simulink library "inverter_loop_pump_and_fan_PWM_LVLibrary"  (R2020a)
settings: Solver=ode45  StartTime=0.0  StopTime=10.0  RelTol=1e-3  EnableMultiTasking=on
undefined symbols (not defined in the file): CR
libraries: simulink x6
settings Model: Creator=aldernl  LastModifiedBy=Harjot
settings DataIOCC: LimitDataPoints=on
settings OptimizationCC: LifeSpan=inf
settings DebuggingCC: AllowSymbolicDim=off  SFUnexpectedBacktrackingDiag=warning  SFNoUnconditionalDefaultTransitionDiag=warning  ArithmeticOperatorsInVariantConditions=warning
settings SFSimCC: SimUseLocalCustomCode=off  CustomCodeUndefinedFunction=UseInterfaceOnly
settings RTWCC: RTWUseLocalCustomCode=off
settings CodeAppCC: StateflowObjectComments=on
settings GRTTargetCC: TargetLangStandard=C89/C90 (ANSI)
settings ConfigComp: CovMetricSettings=dw  CovHtmlReporting=on  CovSaveCumulativeToWorkspaceVar=on  CovSaveSingleToWorkspaceVar=on  CovExternalEMLEnable=off

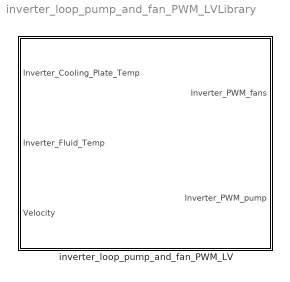
== system inverter_loop_pump_and_fan_PWM_LVLibrary ==
  inverter_loop_pump_and_fan_PWM_LV : Subsystem

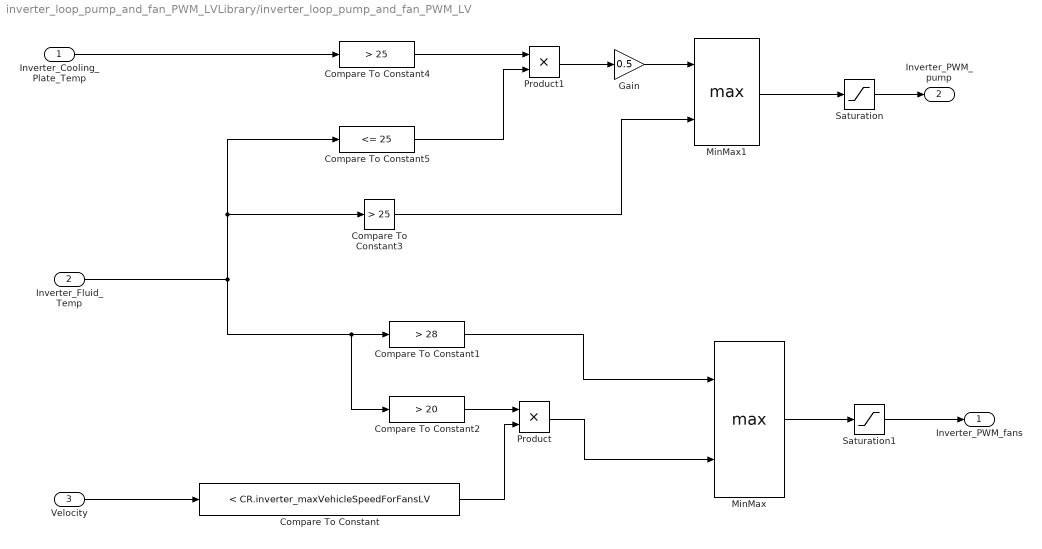
== system inverter_loop_pump_and_fan_PWM_LVLibrary/inverter_loop_pump_and_fan_PWM_LV ==
  Inverter_Cooling_Plate_Temp : Inport  OutDataTypeStr=double  PortDimensions=1
  Inverter_Fluid_Temp : Inport  Port=2  OutDataTypeStr=double  PortDimensions=1
  Velocity : Inport  Port=3  OutDataTypeStr=double  PortDimensions=1
  Compare To Constant : simulink/Logic and Bit Operations/Compare To Constant  relop=<  const=CR.inverter_maxVehicleSpeedForFansLV  OutDataTypeStr=uint8
  Compare To Constant1 : simulink/Logic and Bit Operations/Compare To Constant  relop=>  const=28  OutDataTypeStr=uint8
  Compare To Constant2 : simulink/Logic and Bit Operations/Compare To Constant  relop=>  const=20  OutDataTypeStr=uint8
  Compare To Constant3 : simulink/Logic and Bit Operations/Compare To Constant  relop=>  const=25  OutDataTypeStr=uint8
  Compare To Constant4 : simulink/Logic and Bit Operations/Compare To Constant  relop=>  const=25  OutDataTypeStr=uint8
  Compare To Constant5 : simulink/Logic and Bit Operations/Compare To Constant  relop=<=  const=25  OutDataTypeStr=uint8
  Gain : Gain  Gain=0.5
  MinMax : MinMax  Function=max  Inputs=2  OutDataTypeStr=double
  MinMax1 : MinMax  Function=max  Inputs=2  OutDataTypeStr=double
  Product : Product
  Product1 : Product
  Saturation : Saturate  UpperLimit=CR.inverter_pump_saturation_LV  LowerLimit=0
  Saturation1 : Saturate  UpperLimit=CR.inverter_fan_saturation_LV  LowerLimit=0
  Inverter_PWM_fans : Outport  VectorParamsAs1DForOutWhenUnconnected=off
  Inverter_PWM_pump : Outport  Port=2  VectorParamsAs1DForOutWhenUnconnected=off
  wires:
  Saturation/1 -> Inverter_PWM_pump/1
  Saturation1/1 -> Inverter_PWM_fans/1
  Compare To Constant3/1 -> MinMax1/2
  Gain/1 -> MinMax1/1
  Velocity/1 -> Compare To Constant/1
  Inverter_Fluid_Temp/1 -> Compare To Constant2/1, Compare To Constant1/1, Compare To Constant3/1, Compare To Constant5/1
  Compare To Constant1/1 -> MinMax/1
  Compare To Constant2/1 -> Product/1
  Compare To Constant/1 -> Product/2
  Product/1 -> MinMax/2
  Inverter_Cooling_Plate_Temp/1 -> Compare To Constant4/1
  Compare To Constant5/1 -> Product1/2
  Compare To Constant4/1 -> Product1/1
  Product1/1 -> Gain/1
  MinMax1/1 -> Saturation/1
  MinMax/1 -> Saturation1/1
